simulink model "V2x_TC_CarBreakdownWarning_cs"  (Simulink 7.6)
settings: Solver=ode5  SolverMode=SingleTasking  StartTime=0.0  StopTime=18  FixedStep=1/100  RelTol=1e-3
PreLoadFcn:
  | check_NUTS_defined;
  | 
  | assignin('base',['model_closed_' bdroot],false);addpath('../includes_V2x');
InitFcn:
  | PreScanExperimentInitFcn(bdroot)
StopFcn:
  | PreScanExperimentStopFcn(bdroot)
undefined symbols (not defined in the file or in its folder): acceleration, actorID, actorType, DiscIntNeverNeededParam, GPS_alt, GPS_lat, GPS_long, intmax, lightBarInUse, messageID, Newton, publicActorType, Raphson, rotZ, sigbuilder_block, sireneInUse, trafficLightPriority, turnAdvice, velocity, x_ini_VRML, y_ini_VRML, yawRate, z_ini_VRML
libraries: simulink x61, PreScanSimulinkLibrary x19, PreScanUsefulBlocks x7, simulink_extras x1
(part 9 of 10)

== system V2x_TC_CarBreakdownWarning_cs/Audi_A8_1/Traffic Controller/Traffic signs and  traffic lights controller/Enabled Subsystem ==
  trafficSignType : Inport
  trafficLightsType : Inport  Port=2
  hostRotZ : Inport  Port=3
  hostVelocity : Inport  Port=4
  messageID : Inport  Port=5
  trafficLightPriority : Inport  Port=6
  rotZ : Inport  Port=7
  host GPS lat [deg] : Inport  Port=8
  host GPS long [deg] : Inport  Port=9
  host GPS alt [m] : Inport  Port=10
  GPS_lat : Inport  Port=11
  GPS_long : Inport  Port=12
  GPS_alt : Inport  Port=13
  Enable : EnablePort  StatesWhenEnabling=reset  PropagateVarSize=During execution
  GPS to XYZ difference (vectorized) : Subsystem
  Logical Operator : Logic  AllPortsSameDT=off  OutDataTypeStr=boolean
  Logical Operator1 : Logic  AllPortsSameDT=off  OutDataTypeStr=boolean
  Logical Operator2 : Logic  Inputs=4  AllPortsSameDT=off  OutDataTypeStr=boolean
  distance condition : Subsystem
  heading condition : Subsystem
  hostVelocity1 : InportShadow  Port=4
  major object selection lights : Subsystem
  major object selection signs : Subsystem
  orientation condition : Subsystem
  right road side condition : Subsystem
  signsWarning : Outport
  signsMessage : Outport  Port=2  InitialOutput=0
  lightsWarning : Outport  Port=3
  ligtsMessage : Outport  Port=4  InitialOutput=0
  ligtsPriority : Outport  Port=5  InitialOutput=0
  wires:
  GPS to XYZ difference (vectorized)/3(dY) -> right road side condition/3(dY), orientation condition/3(dY)
  right road side condition/1(orient_cond) -> Logical Operator2/4
  GPS to XYZ difference (vectorized)/1(dist_sq) -> distance condition/1(distance_squared)
  GPS to XYZ difference (vectorized)/2(dX) -> orientation condition/2(dX), right road side condition/2(dX)
  GPS to XYZ difference (vectorized)/4(dZ) -> orientation condition/4(dZ)
  GPS_alt/1 -> GPS to XYZ difference (vectorized)/6(alt)
  orientation condition/1(orient_cond) -> Logical Operator2/3
  GPS_long/1 -> GPS to XYZ difference (vectorized)/5(long)
  GPS_lat/1 -> GPS to XYZ difference (vectorized)/4(lat)
  host GPS alt [m]/1 -> GPS to XYZ difference (vectorized)/3(hostAlt)
  host GPS long [deg]/1 -> GPS to XYZ difference (vectorized)/2(hostLong)
  host GPS lat [deg]/1 -> GPS to XYZ difference (vectorized)/1(hostLat)
  hostVelocity1/1 -> major object selection signs/2(hostVelocity)
  major object selection lights/3(Priority) -> ligtsPriority/1
  major object selection lights/2(MessageID) -> ligtsMessage/1
  major object selection lights/1(Warning) -> lightsWarning/1
  trafficLightPriority/1 -> major object selection lights/3(traffic lights priorities)
  Logical Operator1/1 -> major object selection lights/1(conditions)
  major object selection signs/2(MessageID) -> signsMessage/1
  major object selection signs/1(Warning) -> signsWarning/1
  messageID/1 -> major object selection lights/2(messagesID), major object selection signs/3(messagesID)
  Logical Operator/1 -> major object selection signs/1(conditions)
  trafficLightsType/1 -> Logical Operator1/2
  trafficSignType/1 -> Logical Operator/2
  Logical Operator2/1 -> Logical Operator1/1, Logical Operator/1
  heading condition/1(head_cond) -> Logical Operator2/2
  distance condition/1(dist_cond) -> Logical Operator2/1
  hostRotZ/1 -> orientation condition/1(hostRotZ), right road side condition/1(hostRotZ), heading condition/1(hostRotZ)
  hostVelocity/1 -> distance condition/2(hostVelocity)
  rotZ/1 -> heading condition/2(rotZ)

== system V2x_TC_CarBreakdownWarning_cs/Audi_A8_1/Trajectories/Traj2State1/Traj2State2 ==
  traj : Inport
  MuxState : Subsystem
  Traj2MuxState_Ext : Subsystem
  state : Outport
  wires:
  Traj2MuxState_Ext/9(Y [rad]) -> MuxState/9(Y [rad])
  Traj2MuxState_Ext/8(P [rad]) -> MuxState/8(P [rad])
  Traj2MuxState_Ext/7(R [rad]) -> MuxState/7(R [rad])
  Traj2MuxState_Ext/6(dz [m/s]) -> MuxState/6(dz [m/s])
  Traj2MuxState_Ext/5(dy [m/s]) -> MuxState/5(dy [m/s])
  Traj2MuxState_Ext/4(dx [m/s]) -> MuxState/4(dx [m/s])
  Traj2MuxState_Ext/3(z [m]) -> MuxState/3(z [m])
  Traj2MuxState_Ext/2(y [m]) -> MuxState/2(y [m])
  Traj2MuxState_Ext/1(x [m]) -> MuxState/1(x [m])
  MuxState/1(state) -> state/1
  traj/1 -> Traj2MuxState_Ext/1(Traj)

== system V2x_TC_CarBreakdownWarning_cs/Audi_A8_1/Trajectories/Traj2State2/Traj2State2 ==
  traj : Inport
  MuxState : Subsystem
  Traj2MuxState_Ext : Subsystem
  state : Outport
  wires:
  Traj2MuxState_Ext/9(Y [rad]) -> MuxState/9(Y [rad])
  Traj2MuxState_Ext/8(P [rad]) -> MuxState/8(P [rad])
  Traj2MuxState_Ext/7(R [rad]) -> MuxState/7(R [rad])
  Traj2MuxState_Ext/6(dz [m/s]) -> MuxState/6(dz [m/s])
  Traj2MuxState_Ext/5(dy [m/s]) -> MuxState/5(dy [m/s])
  Traj2MuxState_Ext/4(dx [m/s]) -> MuxState/4(dx [m/s])
  Traj2MuxState_Ext/3(z [m]) -> MuxState/3(z [m])
  Traj2MuxState_Ext/2(y [m]) -> MuxState/2(y [m])
  Traj2MuxState_Ext/1(x [m]) -> MuxState/1(x [m])
  MuxState/1(state) -> state/1
  traj/1 -> Traj2MuxState_Ext/1(Traj)

== system V2x_TC_CarBreakdownWarning_cs/Audi_A8_1/vehicle CAM generator/CAM generation/maybe ==
  x [m] : Inport
  y [m] : Inport  Port=2
  z [m] : Inport  Port=3
  rotZ [deg] : Inport  Port=4
  velocity [m/s] : Inport  Port=5
  Action Port : ActionPort  PropagateVarSize=During execution  ActionType=else
  Add{,1..4} (5 alike) : Sum  Inputs=+-
  Add5 : Sum  Inputs=+++
  Compare To Constant : simulink/Logic and Bit Operations/Compare To Constant  SystemSampleTime=-1  relop=>  const=1  LogicOutDataTypeMode=uint8  ZeroCross=off
  Compare To Constant1 : simulink/Logic and Bit Operations/Compare To Constant  SystemSampleTime=-1  relop=>  const=4  LogicOutDataTypeMode=uint8  ZeroCross=off
  Compare To Constant2 : simulink/Logic and Bit Operations/Compare To Constant  SystemSampleTime=-1  relop=>  const=5^2  LogicOutDataTypeMode=uint8  ZeroCross=off
  Data Store Read : DataStoreRead  DataStoreName=CAM_velocity  SampleTime=0.01
  Data Store Read1 : DataStoreRead  DataStoreName=CAM_heading  SampleTime=0.01
  Data Store Read2 : DataStoreRead  DataStoreName=CAM_x  SampleTime=0.01
  Data Store Read3 : DataStoreRead  DataStoreName=CAM_y  SampleTime=0.01
  Data Store Read4 : DataStoreRead  DataStoreName=CAM_z  SampleTime=0.01
  If : If  IfExpression=u1
  If Action Subsystem : Subsystem  TreatAsAtomicUnit=on
  If Action Subsystem1 : Subsystem  TreatAsAtomicUnit=on
  Logical Operator : Logic  Operator=OR  Inputs=3  AllPortsSameDT=off  OutDataTypeStr=boolean
  Merge : Merge
  Product : Product  RndMeth=Zero
  Product1 : Product  RndMeth=Zero
  Product2 : Product  RndMeth=Zero
  rotZ [deg]1 : InportShadow  Port=4
  velocity [m/s]1 : InportShadow  Port=5
  x [m]1 : InportShadow  Port=1
  y [m]1 : InportShadow  Port=2
  z [m]1 : InportShadow  Port=3
  Out1 : Outport  OutputWhenDisabled=reset  InitialOutput=0
  wires:
  velocity [m/s]/1 -> Add/1
  Data Store Read/1 -> Add/2
  Add/1 -> Compare To Constant/1
  Add1/1 -> Compare To Constant1/1
  rotZ [deg]/1 -> Add1/1
  Data Store Read1/1 -> Add1/2
  x [m]/1 -> Add3/1
  Data Store Read2/1 -> Add3/2
  y [m]/1 -> Add2/1
  Data Store Read3/1 -> Add2/2
  z [m]/1 -> Add4/1
  Data Store Read4/1 -> Add4/2
  Add4/1 -> Product2/2, Product2/1
  Add2/1 -> Product1/2, Product1/1
  Add3/1 -> Product/2, Product/1
  Product/1 -> Add5/1
  Product1/1 -> Add5/2
  Product2/1 -> Add5/3
  Add5/1 -> Compare To Constant2/1
  Compare To Constant/1 -> Logical Operator/1
  Compare To Constant1/1 -> Logical Operator/2
  Compare To Constant2/1 -> Logical Operator/3
  Logical Operator/1 -> If/1
  If/1 -> If Action Subsystem/Action
  If/2 -> If Action Subsystem1/Action
  If Action Subsystem/1(Out1) -> Merge/1
  If Action Subsystem1/1(Out1) -> Merge/2
  Merge/1 -> Out1/1
  x [m]1/1 -> If Action Subsystem/1(x [m])
  y [m]1/1 -> If Action Subsystem/2(y [m])
  z [m]1/1 -> If Action Subsystem/3(z [m])
  rotZ [deg]1/1 -> If Action Subsystem/4(rotZ [deg])
  velocity [m/s]1/1 -> If Action Subsystem/5(velocity [m/s])

== system V2x_TC_CarBreakdownWarning_cs/Audi_A8_1/vehicle CAM generator/CAM generation/no ==
  Action Port : ActionPort  PropagateVarSize=During execution  ActionType=elseif
  Constant : Constant  Value=0
  Out1 : Outport  OutputWhenDisabled=reset  InitialOutput=0
  wires:
  Constant/1 -> Out1/1

== system V2x_TC_CarBreakdownWarning_cs/Audi_A8_1/vehicle CAM generator/CAM generation/yes ==
  x [m] : Inport
  y [m] : Inport  Port=2
  z [m] : Inport  Port=3
  rotZ [deg] : Inport  Port=4
  velocity [m/s] : Inport  Port=5
  Action Port : ActionPort  PropagateVarSize=During execution  ActionType=then
  Constant : Constant
  Data Store Write : DataStoreWrite  DataStoreName=CAM_velocity
  Data Store Write1 : DataStoreWrite  DataStoreName=CAM_heading
  Data Store Write2 : DataStoreWrite  DataStoreName=CAM_x
  Data Store Write3 : DataStoreWrite  DataStoreName=CAM_y
  Data Store Write4 : DataStoreWrite  DataStoreName=CAM_z
  Data Store Write5 : DataStoreWrite  DataStoreName=CAM_time
  Digital Clock1 : DigitalClock  SampleTime=0.01
  Out1 : Outport  OutputWhenDisabled=reset  InitialOutput=0
  wires:
  Constant/1 -> Out1/1
  velocity [m/s]/1 -> Data Store Write/1
  rotZ [deg]/1 -> Data Store Write1/1
  x [m]/1 -> Data Store Write2/1
  y [m]/1 -> Data Store Write3/1
  z [m]/1 -> Data Store Write4/1
  Digital Clock1/1 -> Data Store Write5/1

== system V2x_TC_CarBreakdownWarning_cs/Audi_A8_1/vehicle CAM generator/Subsystem/GPS Noise ==
  GPS_Noise_src : Inport
  Band-Limited White Noise1 : simulink/Sources/Band-Limited White Noise  SystemSampleTime=-1  Cov=1.7  Ts=0.01  seed=randi(intmax, 1)
  Constant : Constant  Value=1/(360*44)
  Product : Product  Inputs=3  RndMeth=Zero
  GPS_Noise : Outport
  wires:
  GPS_Noise_src/1 -> Product/1
  Band-Limited White Noise1/1 -> Product/2
  Constant/1 -> Product/3
  Product/1 -> GPS_Noise/1

== system V2x_TC_CarBreakdownWarning_cs/Audi_A8_1/vehicle CAM generator/Subsystem1/GPS Noise ==
  GPS_Noise_src : Inport
  Band-Limited White Noise1 : simulink/Sources/Band-Limited White Noise  SystemSampleTime=-1  Cov=1.7  Ts=0.01  seed=randi(intmax, 1)
  Constant : Constant  Value=1/(360*44)
  Product : Product  Inputs=3  RndMeth=Zero
  GPS_Noise : Outport
  wires:
  Product/1 -> GPS_Noise/1
  Constant/1 -> Product/3
  Band-Limited White Noise1/1 -> Product/2
  GPS_Noise_src/1 -> Product/1

== system V2x_TC_CarBreakdownWarning_cs/Audi_A8_1/vehicle CAM generator/Subsystem2/GPS Noise ==
  GPS_Noise_src : Inport
  Band-Limited White Noise1 : simulink/Sources/Band-Limited White Noise  SystemSampleTime=-1  Cov=1.7  Ts=0.01  seed=randi(intmax, 1)
  Constant : Constant  Value=1/(360*44)
  Product : Product  Inputs=3  RndMeth=Zero
  GPS_Noise : Outport
  wires:
  GPS_Noise_src/1 -> Product/1
  Band-Limited White Noise1/1 -> Product/2
  Constant/1 -> Product/3
  Product/1 -> GPS_Noise/1

== system V2x_TC_CarBreakdownWarning_cs/Audi_A8_1/vehicle CAM generator/Subsystem3/GPS Noise ==
  GPS_Noise_src : Inport
  Band-Limited White Noise1 : simulink/Sources/Band-Limited White Noise  SystemSampleTime=-1  Cov=1.7  Ts=0.01  seed=randi(intmax, 1)
  Constant : Constant  Value=1/(360*44)
  Product : Product  Inputs=3  RndMeth=Zero
  GPS_Noise : Outport
  wires:
  Product/1 -> GPS_Noise/1
  Constant/1 -> Product/3
  Band-Limited White Noise1/1 -> Product/2
  GPS_Noise_src/1 -> Product/1

== system V2x_TC_CarBreakdownWarning_cs/BMW_X5_1/SELF_Demux/compas converter/cart2compas ==
  Angle [deg] : Inport
  Constant : Constant  Value=90
  Constant1 : Constant  Value=360
  Gain : Gain  Gain=1/360
  Gain1 : Gain  Gain=360
  Gain2 : Gain  Gain=-1
  Rounding Function : Rounding
  Sum : Sum  Inputs=|-+
  Sum1 : Sum  Inputs=-+|
  Sum2 : Sum  Inputs=++|
  heading [deg] : Outport
  wires:
  Sum2/1 -> heading [deg]/1
  Constant1/1 -> Sum2/1
  Gain2/1 -> Sum2/2
  Constant/1 -> Sum1/1
  Sum1/1 -> Sum/2, Gain/1
  Sum/1 -> Gain2/1
  Angle [deg]/1 -> Sum1/2
  Gain1/1 -> Sum/1
  Rounding Function/1 -> Gain1/1
  Gain/1 -> Rounding Function/1

== system V2x_TC_CarBreakdownWarning_cs/BMW_X5_1/Trajectories/Traj2State1/Traj2State2 ==
  traj : Inport
  MuxState : Subsystem
  Traj2MuxState_Ext : Subsystem
  state : Outport
  wires:
  Traj2MuxState_Ext/9(Y [rad]) -> MuxState/9(Y [rad])
  Traj2MuxState_Ext/8(P [rad]) -> MuxState/8(P [rad])
  Traj2MuxState_Ext/7(R [rad]) -> MuxState/7(R [rad])
  Traj2MuxState_Ext/6(dz [m/s]) -> MuxState/6(dz [m/s])
  Traj2MuxState_Ext/5(dy [m/s]) -> MuxState/5(dy [m/s])
  Traj2MuxState_Ext/4(dx [m/s]) -> MuxState/4(dx [m/s])
  Traj2MuxState_Ext/3(z [m]) -> MuxState/3(z [m])
  Traj2MuxState_Ext/2(y [m]) -> MuxState/2(y [m])
  Traj2MuxState_Ext/1(x [m]) -> MuxState/1(x [m])
  MuxState/1(state) -> state/1
  traj/1 -> Traj2MuxState_Ext/1(Traj)

== system V2x_TC_CarBreakdownWarning_cs/BMW_X5_1/vehicle CAM generator/CAM generation/maybe ==
  x [m] : Inport
  y [m] : Inport  Port=2
  z [m] : Inport  Port=3
  rotZ [deg] : Inport  Port=4
  velocity [m/s] : Inport  Port=5
  Action Port : ActionPort  PropagateVarSize=During execution  ActionType=else
  Add{,1..4} (5 alike) : Sum  Inputs=+-
  Add5 : Sum  Inputs=+++
  Compare To Constant : simulink/Logic and Bit Operations/Compare To Constant  SystemSampleTime=-1  relop=>  const=1  LogicOutDataTypeMode=uint8  ZeroCross=off
  Compare To Constant1 : simulink/Logic and Bit Operations/Compare To Constant  SystemSampleTime=-1  relop=>  const=4  LogicOutDataTypeMode=uint8  ZeroCross=off
  Compare To Constant2 : simulink/Logic and Bit Operations/Compare To Constant  SystemSampleTime=-1  relop=>  const=5^2  LogicOutDataTypeMode=uint8  ZeroCross=off
  Data Store Read : DataStoreRead  DataStoreName=CAM_velocity  SampleTime=0.01
  Data Store Read1 : DataStoreRead  DataStoreName=CAM_heading  SampleTime=0.01
  Data Store Read2 : DataStoreRead  DataStoreName=CAM_x  SampleTime=0.01
  Data Store Read3 : DataStoreRead  DataStoreName=CAM_y  SampleTime=0.01
  Data Store Read4 : DataStoreRead  DataStoreName=CAM_z  SampleTime=0.01
  If : If  IfExpression=u1
  If Action Subsystem : Subsystem  TreatAsAtomicUnit=on
  If Action Subsystem1 : Subsystem  TreatAsAtomicUnit=on
  Logical Operator : Logic  Operator=OR  Inputs=3  AllPortsSameDT=off  OutDataTypeStr=boolean
  Merge : Merge
  Product : Product  RndMeth=Zero
  Product1 : Product  RndMeth=Zero
  Product2 : Product  RndMeth=Zero
  rotZ [deg]1 : InportShadow  Port=4
  velocity [m/s]1 : InportShadow  Port=5
  x [m]1 : InportShadow  Port=1
  y [m]1 : InportShadow  Port=2
  z [m]1 : InportShadow  Port=3
  Out1 : Outport  OutputWhenDisabled=reset  InitialOutput=0
  wires:
  velocity [m/s]/1 -> Add/1
  Data Store Read/1 -> Add/2
  Add/1 -> Compare To Constant/1
  Add1/1 -> Compare To Constant1/1
  rotZ [deg]/1 -> Add1/1
  Data Store Read1/1 -> Add1/2
  x [m]/1 -> Add3/1
  Data Store Read2/1 -> Add3/2
  y [m]/1 -> Add2/1
  Data Store Read3/1 -> Add2/2
  z [m]/1 -> Add4/1
  Data Store Read4/1 -> Add4/2
  Add4/1 -> Product2/2, Product2/1
  Add2/1 -> Product1/2, Product1/1
  Add3/1 -> Product/2, Product/1
  Product/1 -> Add5/1
  Product1/1 -> Add5/2
  Product2/1 -> Add5/3
  Add5/1 -> Compare To Constant2/1
  Compare To Constant/1 -> Logical Operator/1
  Compare To Constant1/1 -> Logical Operator/2
  Compare To Constant2/1 -> Logical Operator/3
  Logical Operator/1 -> If/1
  If/1 -> If Action Subsystem/Action
  If/2 -> If Action Subsystem1/Action
  If Action Subsystem/1(Out1) -> Merge/1
  If Action Subsystem1/1(Out1) -> Merge/2
  Merge/1 -> Out1/1
  x [m]1/1 -> If Action Subsystem/1(x [m])
  y [m]1/1 -> If Action Subsystem/2(y [m])
  z [m]1/1 -> If Action Subsystem/3(z [m])
  rotZ [deg]1/1 -> If Action Subsystem/4(rotZ [deg])
  velocity [m/s]1/1 -> If Action Subsystem/5(velocity [m/s])

== system V2x_TC_CarBreakdownWarning_cs/BMW_X5_1/vehicle CAM generator/CAM generation/no ==
  Action Port : ActionPort  PropagateVarSize=During execution  ActionType=elseif
  Constant : Constant  Value=0
  Out1 : Outport  OutputWhenDisabled=reset  InitialOutput=0
  wires:
  Constant/1 -> Out1/1

== system V2x_TC_CarBreakdownWarning_cs/BMW_X5_1/vehicle CAM generator/CAM generation/yes ==
  x [m] : Inport
  y [m] : Inport  Port=2
  z [m] : Inport  Port=3
  rotZ [deg] : Inport  Port=4
  velocity [m/s] : Inport  Port=5
  Action Port : ActionPort  PropagateVarSize=During execution  ActionType=then
  Constant : Constant
  Data Store Write : DataStoreWrite  DataStoreName=CAM_velocity
  Data Store Write1 : DataStoreWrite  DataStoreName=CAM_heading
  Data Store Write2 : DataStoreWrite  DataStoreName=CAM_x
  Data Store Write3 : DataStoreWrite  DataStoreName=CAM_y
  Data Store Write4 : DataStoreWrite  DataStoreName=CAM_z
  Data Store Write5 : DataStoreWrite  DataStoreName=CAM_time
  Digital Clock1 : DigitalClock  SampleTime=0.01
  Out1 : Outport  OutputWhenDisabled=reset  InitialOutput=0
  wires:
  Constant/1 -> Out1/1
  velocity [m/s]/1 -> Data Store Write/1
  rotZ [deg]/1 -> Data Store Write1/1
  x [m]/1 -> Data Store Write2/1
  y [m]/1 -> Data Store Write3/1
  z [m]/1 -> Data Store Write4/1
  Digital Clock1/1 -> Data Store Write5/1

== system V2x_TC_CarBreakdownWarning_cs/CameraTrolley/SELF_Demux/compas converter/cart2compas ==
  Angle [deg] : Inport
  Constant : Constant  Value=90
  Constant1 : Constant  Value=360
  Gain : Gain  Gain=1/360
  Gain1 : Gain  Gain=360
  Gain2 : Gain  Gain=-1
  Rounding Function : Rounding
  Sum : Sum  Inputs=|-+
  Sum1 : Sum  Inputs=-+|
  Sum2 : Sum  Inputs=++|
  heading [deg] : Outport
  wires:
  Sum2/1 -> heading [deg]/1
  Constant1/1 -> Sum2/1
  Gain2/1 -> Sum2/2
  Constant/1 -> Sum1/1
  Sum1/1 -> Sum/2, Gain/1
  Sum/1 -> Gain2/1
  Angle [deg]/1 -> Sum1/2
  Gain1/1 -> Sum/1
  Rounding Function/1 -> Gain1/1
  Gain/1 -> Rounding Function/1

== system V2x_TC_CarBreakdownWarning_cs/Fiat_Bravo_1/SELF_Demux/compas converter/cart2compas ==
  Angle [deg] : Inport
  Constant : Constant  Value=90
  Constant1 : Constant  Value=360
  Gain : Gain  Gain=1/360
  Gain1 : Gain  Gain=360
  Gain2 : Gain  Gain=-1
  Rounding Function : Rounding
  Sum : Sum  Inputs=|-+
  Sum1 : Sum  Inputs=-+|
  Sum2 : Sum  Inputs=++|
  heading [deg] : Outport
  wires:
  Sum2/1 -> heading [deg]/1
  Constant1/1 -> Sum2/1
  Gain2/1 -> Sum2/2
  Constant/1 -> Sum1/1
  Sum1/1 -> Sum/2, Gain/1
  Sum/1 -> Gain2/1
  Angle [deg]/1 -> Sum1/2
  Gain1/1 -> Sum/1
  Rounding Function/1 -> Gain1/1
  Gain/1 -> Rounding Function/1

== system V2x_TC_CarBreakdownWarning_cs/Fiat_Bravo_1/Trajectories/Traj2State1/Traj2State2 ==
  traj : Inport
  MuxState : Subsystem
  Traj2MuxState_Ext : Subsystem
  state : Outport
  wires:
  Traj2MuxState_Ext/9(Y [rad]) -> MuxState/9(Y [rad])
  Traj2MuxState_Ext/8(P [rad]) -> MuxState/8(P [rad])
  Traj2MuxState_Ext/7(R [rad]) -> MuxState/7(R [rad])
  Traj2MuxState_Ext/6(dz [m/s]) -> MuxState/6(dz [m/s])
  Traj2MuxState_Ext/5(dy [m/s]) -> MuxState/5(dy [m/s])
  Traj2MuxState_Ext/4(dx [m/s]) -> MuxState/4(dx [m/s])
  Traj2MuxState_Ext/3(z [m]) -> MuxState/3(z [m])
  Traj2MuxState_Ext/2(y [m]) -> MuxState/2(y [m])
  Traj2MuxState_Ext/1(x [m]) -> MuxState/1(x [m])
  MuxState/1(state) -> state/1
  traj/1 -> Traj2MuxState_Ext/1(Traj)

== system V2x_TC_CarBreakdownWarning_cs/Fiat_Bravo_1/vehicle CAM generator/CAM generation/maybe ==
  x [m] : Inport
  y [m] : Inport  Port=2
  z [m] : Inport  Port=3
  rotZ [deg] : Inport  Port=4
  velocity [m/s] : Inport  Port=5
  Action Port : ActionPort  PropagateVarSize=During execution  ActionType=else
  Add{,1..4} (5 alike) : Sum  Inputs=+-
  Add5 : Sum  Inputs=+++
  Compare To Constant : simulink/Logic and Bit Operations/Compare To Constant  SystemSampleTime=-1  relop=>  const=1  LogicOutDataTypeMode=uint8  ZeroCross=off
  Compare To Constant1 : simulink/Logic and Bit Operations/Compare To Constant  SystemSampleTime=-1  relop=>  const=4  LogicOutDataTypeMode=uint8  ZeroCross=off
  Compare To Constant2 : simulink/Logic and Bit Operations/Compare To Constant  SystemSampleTime=-1  relop=>  const=5^2  LogicOutDataTypeMode=uint8  ZeroCross=off
  Data Store Read : DataStoreRead  DataStoreName=CAM_velocity  SampleTime=0.01
  Data Store Read1 : DataStoreRead  DataStoreName=CAM_heading  SampleTime=0.01
  Data Store Read2 : DataStoreRead  DataStoreName=CAM_x  SampleTime=0.01
  Data Store Read3 : DataStoreRead  DataStoreName=CAM_y  SampleTime=0.01
  Data Store Read4 : DataStoreRead  DataStoreName=CAM_z  SampleTime=0.01
  If : If  IfExpression=u1
  If Action Subsystem : Subsystem  TreatAsAtomicUnit=on
  If Action Subsystem1 : Subsystem  TreatAsAtomicUnit=on
  Logical Operator : Logic  Operator=OR  Inputs=3  AllPortsSameDT=off  OutDataTypeStr=boolean
  Merge : Merge
  Product : Product  RndMeth=Zero
  Product1 : Product  RndMeth=Zero
  Product2 : Product  RndMeth=Zero
  rotZ [deg]1 : InportShadow  Port=4
  velocity [m/s]1 : InportShadow  Port=5
  x [m]1 : InportShadow  Port=1
  y [m]1 : InportShadow  Port=2
  z [m]1 : InportShadow  Port=3
  Out1 : Outport  OutputWhenDisabled=reset  InitialOutput=0
  wires:
  velocity [m/s]/1 -> Add/1
  Data Store Read/1 -> Add/2
  Add/1 -> Compare To Constant/1
  Add1/1 -> Compare To Constant1/1
  rotZ [deg]/1 -> Add1/1
  Data Store Read1/1 -> Add1/2
  x [m]/1 -> Add3/1
  Data Store Read2/1 -> Add3/2
  y [m]/1 -> Add2/1
  Data Store Read3/1 -> Add2/2
  z [m]/1 -> Add4/1
  Data Store Read4/1 -> Add4/2
  Add4/1 -> Product2/2, Product2/1
  Add2/1 -> Product1/2, Product1/1
  Add3/1 -> Product/2, Product/1
  Product/1 -> Add5/1
  Product1/1 -> Add5/2
  Product2/1 -> Add5/3
  Add5/1 -> Compare To Constant2/1
  Compare To Constant/1 -> Logical Operator/1
  Compare To Constant1/1 -> Logical Operator/2
  Compare To Constant2/1 -> Logical Operator/3
  Logical Operator/1 -> If/1
  If/1 -> If Action Subsystem/Action
  If/2 -> If Action Subsystem1/Action
  If Action Subsystem/1(Out1) -> Merge/1
  If Action Subsystem1/1(Out1) -> Merge/2
  Merge/1 -> Out1/1
  x [m]1/1 -> If Action Subsystem/1(x [m])
  y [m]1/1 -> If Action Subsystem/2(y [m])
  z [m]1/1 -> If Action Subsystem/3(z [m])
  rotZ [deg]1/1 -> If Action Subsystem/4(rotZ [deg])
  velocity [m/s]1/1 -> If Action Subsystem/5(velocity [m/s])

== system V2x_TC_CarBreakdownWarning_cs/Fiat_Bravo_1/vehicle CAM generator/CAM generation/no ==
  Action Port : ActionPort  PropagateVarSize=During execution  ActionType=elseif
  Constant : Constant  Value=0
  Out1 : Outport  OutputWhenDisabled=reset  InitialOutput=0
  wires:
  Constant/1 -> Out1/1

== system V2x_TC_CarBreakdownWarning_cs/Fiat_Bravo_1/vehicle CAM generator/CAM generation/yes ==
  x [m] : Inport
  y [m] : Inport  Port=2
  z [m] : Inport  Port=3
  rotZ [deg] : Inport  Port=4
  velocity [m/s] : Inport  Port=5
  Action Port : ActionPort  PropagateVarSize=During execution  ActionType=then
  Constant : Constant
  Data Store Write : DataStoreWrite  DataStoreName=CAM_velocity
  Data Store Write1 : DataStoreWrite  DataStoreName=CAM_heading
  Data Store Write2 : DataStoreWrite  DataStoreName=CAM_x
  Data Store Write3 : DataStoreWrite  DataStoreName=CAM_y
  Data Store Write4 : DataStoreWrite  DataStoreName=CAM_z
  Data Store Write5 : DataStoreWrite  DataStoreName=CAM_time
  Digital Clock1 : DigitalClock  SampleTime=0.01
  Out1 : Outport  OutputWhenDisabled=reset  InitialOutput=0
  wires:
  Constant/1 -> Out1/1
  velocity [m/s]/1 -> Data Store Write/1
  rotZ [deg]/1 -> Data Store Write1/1
  x [m]/1 -> Data Store Write2/1
  y [m]/1 -> Data Store Write3/1
  z [m]/1 -> Data Store Write4/1
  Digital Clock1/1 -> Data Store Write5/1

== system V2x_TC_CarBreakdownWarning_cs/Toyota_Previa_1/Antenna_Rx_1_Demux/compas converter/cart2compas ==
  Angle [deg] : Inport
  Constant : Constant  Value=90
  Constant1 : Constant  Value=360
  Gain : Gain  Gain=1/360
  Gain1 : Gain  Gain=360
  Gain2 : Gain  Gain=-1
  Rounding Function : Rounding
  Sum : Sum  Inputs=|-+
  Sum1 : Sum  Inputs=-+|
  Sum2 : Sum  Inputs=++|
  heading [deg] : Outport
  wires:
  Gain/1 -> Rounding Function/1
  Rounding Function/1 -> Gain1/1
  Gain1/1 -> Sum/1
  Angle [deg]/1 -> Sum1/2
  Sum/1 -> Gain2/1
  Sum1/1 -> Gain/1, Sum/2
  Constant/1 -> Sum1/1
  Gain2/1 -> Sum2/2
  Constant1/1 -> Sum2/1
  Sum2/1 -> heading [deg]/1

== system V2x_TC_CarBreakdownWarning_cs/Toyota_Previa_1/SELF_Demux/compas converter/cart2compas ==
  Angle [deg] : Inport
  Constant : Constant  Value=90
  Constant1 : Constant  Value=360
  Gain : Gain  Gain=1/360
  Gain1 : Gain  Gain=360
  Gain2 : Gain  Gain=-1
  Rounding Function : Rounding
  Sum : Sum  Inputs=|-+
  Sum1 : Sum  Inputs=-+|
  Sum2 : Sum  Inputs=++|
  heading [deg] : Outport
  wires:
  Sum2/1 -> heading [deg]/1
  Constant1/1 -> Sum2/1
  Gain2/1 -> Sum2/2
  Constant/1 -> Sum1/1
  Sum1/1 -> Sum/2, Gain/1
  Sum/1 -> Gain2/1
  Angle [deg]/1 -> Sum1/2
  Gain1/1 -> Sum/1
  Rounding Function/1 -> Gain1/1
  Gain/1 -> Rounding Function/1

== system V2x_TC_CarBreakdownWarning_cs/Toyota_Previa_1/vehicle CAM generator/CAM generation/maybe ==
  x [m] : Inport
  y [m] : Inport  Port=2
  z [m] : Inport  Port=3
  rotZ [deg] : Inport  Port=4
  velocity [m/s] : Inport  Port=5
  Action Port : ActionPort  PropagateVarSize=During execution  ActionType=else
  Add{,1..4} (5 alike) : Sum  Inputs=+-
  Add5 : Sum  Inputs=+++
  Compare To Constant : simulink/Logic and Bit Operations/Compare To Constant  SystemSampleTime=-1  relop=>  const=1  LogicOutDataTypeMode=uint8  ZeroCross=off
  Compare To Constant1 : simulink/Logic and Bit Operations/Compare To Constant  SystemSampleTime=-1  relop=>  const=4  LogicOutDataTypeMode=uint8  ZeroCross=off
  Compare To Constant2 : simulink/Logic and Bit Operations/Compare To Constant  SystemSampleTime=-1  relop=>  const=5^2  LogicOutDataTypeMode=uint8  ZeroCross=off
  Data Store Read : DataStoreRead  DataStoreName=CAM_velocity  SampleTime=0.01
  Data Store Read1 : DataStoreRead  DataStoreName=CAM_heading  SampleTime=0.01
  Data Store Read2 : DataStoreRead  DataStoreName=CAM_x  SampleTime=0.01
  Data Store Read3 : DataStoreRead  DataStoreName=CAM_y  SampleTime=0.01
  Data Store Read4 : DataStoreRead  DataStoreName=CAM_z  SampleTime=0.01
  If : If  IfExpression=u1
  If Action Subsystem : Subsystem  TreatAsAtomicUnit=on
  If Action Subsystem1 : Subsystem  TreatAsAtomicUnit=on
  Logical Operator : Logic  Operator=OR  Inputs=3  AllPortsSameDT=off  OutDataTypeStr=boolean
  Merge : Merge
  Product : Product  RndMeth=Zero
  Product1 : Product  RndMeth=Zero
  Product2 : Product  RndMeth=Zero
  rotZ [deg]1 : InportShadow  Port=4
  velocity [m/s]1 : InportShadow  Port=5
  x [m]1 : InportShadow  Port=1
  y [m]1 : InportShadow  Port=2
  z [m]1 : InportShadow  Port=3
  Out1 : Outport  OutputWhenDisabled=reset  InitialOutput=0
  wires:
  velocity [m/s]/1 -> Add/1
  Data Store Read/1 -> Add/2
  Add/1 -> Compare To Constant/1
  Add1/1 -> Compare To Constant1/1
  rotZ [deg]/1 -> Add1/1
  Data Store Read1/1 -> Add1/2
  x [m]/1 -> Add3/1
  Data Store Read2/1 -> Add3/2
  y [m]/1 -> Add2/1
  Data Store Read3/1 -> Add2/2
  z [m]/1 -> Add4/1
  Data Store Read4/1 -> Add4/2
  Add4/1 -> Product2/2, Product2/1
  Add2/1 -> Product1/2, Product1/1
  Add3/1 -> Product/2, Product/1
  Product/1 -> Add5/1
  Product1/1 -> Add5/2
  Product2/1 -> Add5/3
  Add5/1 -> Compare To Constant2/1
  Compare To Constant/1 -> Logical Operator/1
  Compare To Constant1/1 -> Logical Operator/2
  Compare To Constant2/1 -> Logical Operator/3
  Logical Operator/1 -> If/1
  If/1 -> If Action Subsystem/Action
  If/2 -> If Action Subsystem1/Action
  If Action Subsystem/1(Out1) -> Merge/1
  If Action Subsystem1/1(Out1) -> Merge/2
  Merge/1 -> Out1/1
  x [m]1/1 -> If Action Subsystem/1(x [m])
  y [m]1/1 -> If Action Subsystem/2(y [m])
  z [m]1/1 -> If Action Subsystem/3(z [m])
  rotZ [deg]1/1 -> If Action Subsystem/4(rotZ [deg])
  velocity [m/s]1/1 -> If Action Subsystem/5(velocity [m/s])

== system V2x_TC_CarBreakdownWarning_cs/Toyota_Previa_1/vehicle CAM generator/CAM generation/no ==
  Action Port : ActionPort  PropagateVarSize=During execution  ActionType=elseif
  Constant : Constant  Value=0
  Out1 : Outport  OutputWhenDisabled=reset  InitialOutput=0
  wires:
  Constant/1 -> Out1/1

== system V2x_TC_CarBreakdownWarning_cs/Toyota_Previa_1/vehicle CAM generator/CAM generation/yes ==
  x [m] : Inport
  y [m] : Inport  Port=2
  z [m] : Inport  Port=3
  rotZ [deg] : Inport  Port=4
  velocity [m/s] : Inport  Port=5
  Action Port : ActionPort  PropagateVarSize=During execution  ActionType=then
  Constant : Constant
  Data Store Write : DataStoreWrite  DataStoreName=CAM_velocity
  Data Store Write1 : DataStoreWrite  DataStoreName=CAM_heading
  Data Store Write2 : DataStoreWrite  DataStoreName=CAM_x
  Data Store Write3 : DataStoreWrite  DataStoreName=CAM_y
  Data Store Write4 : DataStoreWrite  DataStoreName=CAM_z
  Data Store Write5 : DataStoreWrite  DataStoreName=CAM_time
  Digital Clock1 : DigitalClock  SampleTime=0.01
  Out1 : Outport  OutputWhenDisabled=reset  InitialOutput=0
  wires:
  Constant/1 -> Out1/1
  velocity [m/s]/1 -> Data Store Write/1
  rotZ [deg]/1 -> Data Store Write1/1
  x [m]/1 -> Data Store Write2/1
  y [m]/1 -> Data Store Write3/1
  z [m]/1 -> Data Store Write4/1
  Digital Clock1/1 -> Data Store Write5/1

== system V2x_TC_CarBreakdownWarning_cs/Toyota_Previa_1/vehicle CAM generator/Subsystem/GPS Noise ==
  GPS_Noise_src : Inport
  Band-Limited White Noise1 : simulink/Sources/Band-Limited White Noise  SystemSampleTime=-1  Cov=1.7  Ts=0.01  seed=randi(intmax, 1)
  Constant : Constant  Value=1/(360*44)
  Product : Product  Inputs=3  RndMeth=Zero
  GPS_Noise : Outport
  wires:
  GPS_Noise_src/1 -> Product/1
  Band-Limited White Noise1/1 -> Product/2
  Constant/1 -> Product/3
  Product/1 -> GPS_Noise/1

== system V2x_TC_CarBreakdownWarning_cs/Toyota_Previa_1/vehicle CAM generator/Subsystem1/GPS Noise ==
  GPS_Noise_src : Inport
  Band-Limited White Noise1 : simulink/Sources/Band-Limited White Noise  SystemSampleTime=-1  Cov=1.7  Ts=0.01  seed=randi(intmax, 1)
  Constant : Constant  Value=1/(360*44)
  Product : Product  Inputs=3  RndMeth=Zero
  GPS_Noise : Outport
  wires:
  Product/1 -> GPS_Noise/1
  Constant/1 -> Product/3
  Band-Limited White Noise1/1 -> Product/2
  GPS_Noise_src/1 -> Product/1

== system V2x_TC_CarBreakdownWarning_cs/Toyota_Previa_1/vehicle CAM generator/Subsystem2/GPS Noise ==
  GPS_Noise_src : Inport
  Band-Limited White Noise1 : simulink/Sources/Band-Limited White Noise  SystemSampleTime=-1  Cov=1.7  Ts=0.01  seed=randi(intmax, 1)
  Constant : Constant  Value=1/(360*44)
  Product : Product  Inputs=3  RndMeth=Zero
  GPS_Noise : Outport
  wires:
  GPS_Noise_src/1 -> Product/1
  Band-Limited White Noise1/1 -> Product/2
  Constant/1 -> Product/3
  Product/1 -> GPS_Noise/1

== system V2x_TC_CarBreakdownWarning_cs/Toyota_Previa_1/vehicle CAM generator/Subsystem3/GPS Noise ==
  GPS_Noise_src : Inport
  Band-Limited White Noise1 : simulink/Sources/Band-Limited White Noise  SystemSampleTime=-1  Cov=1.7  Ts=0.01  seed=randi(intmax, 1)
  Constant : Constant  Value=1/(360*44)
  Product : Product  Inputs=3  RndMeth=Zero
  GPS_Noise : Outport
  wires:
  Product/1 -> GPS_Noise/1
  Constant/1 -> Product/3
  Band-Limited White Noise1/1 -> Product/2
  GPS_Noise_src/1 -> Product/1

== system V2x_TC_CarBreakdownWarning_cs/Audi_A8_1/Traffic Controller/Intersection warning controller/Enabled Subsystem/Intersection ==
  hostRotZ : Inport
  hostTurnAdvice : Inport  Port=2
  host GPS lat [deg] : Inport  Port=3
  host GPS long [deg] : Inport  Port=4
  host GPS alt [m] : Inport  Port=5
  GPS_lat : Inport  Port=6
  GPS_long : Inport  Port=7
  GPS_alt : Inport  Port=8
  targetVelocity : Inport  Port=9
  turnAdvice : Inport  Port=10
  rotZ : Inport  Port=11
  actorType : Inport  Port=12
  crossingType : Inport  Port=13
  crossing detection range : Inport  Port=14
  Closest crossing selection : Subsystem
  GPS to XYZ difference (vectorized) : Subsystem
  GPS_alt_1 : InportShadow  Port=8
  GPS_lat_1 : InportShadow  Port=6
  GPS_long_1 : InportShadow  Port=7
  Intersection collision warning controller : Subsystem
  Terminator_2 : Terminator
  cartesian 2 cylindrical : Subsystem
  crossing detection range_1 : InportShadow  Port=14
  hostRotZ_1 : InportShadow  Port=1
  relative heading : Subsystem
  warning left lane : Outport
  warning straight lane : Outport  Port=2
  warning right lane : Outport  Port=3
  wires:
  host GPS lat [deg]/1 -> Closest crossing selection/2(host GPS lat)
  host GPS long [deg]/1 -> Closest crossing selection/3(host GPS long)
  host GPS alt [m]/1 -> Closest crossing selection/4(host GPS alt)
  Closest crossing selection/1(crossing GPS lat) -> GPS to XYZ difference (vectorized)/1(hostLat)
  Closest crossing selection/2(crossing GPS long) -> GPS to XYZ difference (vectorized)/2(hostLong)
  Closest crossing selection/3(crossing GPS alt) -> GPS to XYZ difference (vectorized)/3(hostAlt)
  crossing detection range/1 -> Closest crossing selection/8(crossing detection range)
  crossing detection range_1/1 -> Intersection collision warning controller/3(crossing detection range)
  hostRotZ/1 -> relative heading/2(hostRotZ)
  hostTurnAdvice/1 -> Intersection collision warning controller/2(hostTurnAdvice)
  cartesian 2 cylindrical/1(range) -> Intersection collision warning controller/6(target range)
  relative heading/1(dRotZ) -> Intersection collision warning controller/8(target heading)
  Intersection collision warning controller/1(warning left lane) -> warning left lane/1
  Intersection collision warning controller/2(warning straight lane) -> warning straight lane/1
  Intersection collision warning controller/3(warning right lane) -> warning right lane/1
  GPS to XYZ difference (vectorized)/1(dX) -> cartesian 2 cylindrical/1(dX)
  GPS to XYZ difference (vectorized)/2(dY) -> cartesian 2 cylindrical/2(dY)
  GPS_lat/1 -> Closest crossing selection/5(GPS lat)
  GPS_long/1 -> Closest crossing selection/6(GPS long)
  GPS_alt/1 -> Closest crossing selection/7(GPS alt)
  crossingType/1 -> Closest crossing selection/1(crossingType)
  rotZ/1 -> relative heading/1(rotZ)
  GPS_lat_1/1 -> GPS to XYZ difference (vectorized)/4(lat)
  GPS_long_1/1 -> GPS to XYZ difference (vectorized)/5(long)
  GPS_alt_1/1 -> GPS to XYZ difference (vectorized)/6(alt)
  turnAdvice/1 -> Intersection collision warning controller/4(target intention)
  targetVelocity/1 -> Intersection collision warning controller/5(target velocity)
  actorType/1 -> Intersection collision warning controller/1(actorType)
  GPS to XYZ difference (vectorized)/3(dZ) -> Terminator_2/1
  hostRotZ_1/1 -> cartesian 2 cylindrical/3(hostRotZ)
  cartesian 2 cylindrical/2(angle) -> Intersection collision warning controller/7(target angle)

== system V2x_TC_CarBreakdownWarning_cs/Audi_A8_1/Traffic Controller/Intersection warning controller/Enabled Subsystem/sort using ID ==
  IDs : Inport
  in1 : Inport  Port=2
  in2 : Inport  Port=3
  in3 : Inport  Port=4
  in4 : Inport  Port=5
  in5 : Inport  Port=6
  in6 : Inport  Port=7
  in7 : Inport  Port=8
  in8 : Inport  Port=9
  Embedded MATLAB Function : Stateflow chart  TreatAsAtomicUnit=on
  Selector{1..8} (8 alike) : Selector  IndexOptions=Index vector (port)  Indices=[1 3]  OutputSizes=1
  Out1 : Outport
  Out2 : Outport  Port=2
  Out3 : Outport  Port=3
  Out4 : Outport  Port=4
  Out5 : Outport  Port=5
  Out6 : Outport  Port=6
  Out7 : Outport  Port=7
  Out8 : Outport  Port=8
  wires:
  Embedded MATLAB Function/1(y) -> Selector7/2, Selector8/2, Selector6/2, Selector5/2, Selector4/2, Selector3/2, Selector2/2, Selector1/2
  IDs/1 -> Embedded MATLAB Function/1(ids)
  in7/1 -> Selector7/1
  in6/1 -> Selector6/1
  Selector7/1 -> Out7/1
  Selector6/1 -> Out6/1
  in5/1 -> Selector5/1
  in4/1 -> Selector4/1
  in3/1 -> Selector3/1
  in2/1 -> Selector2/1
  Selector5/1 -> Out5/1
  Selector4/1 -> Out4/1
  Selector3/1 -> Out3/1
  Selector2/1 -> Out2/1
  Selector1/1 -> Out1/1
  in1/1 -> Selector1/1
  in8/1 -> Selector8/1
  Selector8/1 -> Out8/1

== system V2x_TC_CarBreakdownWarning_cs/Audi_A8_1/Traffic Controller/Road accident detection controller/Compute distance to road accident/If Action Subsystem ==
  conditions : Inport
  GPS lat1 : Inport  Port=2
  GPS long1 : Inport  Port=3
  GPS alt1 : Inport  Port=4
  host_GPS_lat : Inport  Port=5
  host_GPS_long : Inport  Port=6
  host_GPS_alt : Inport  Port=7
  Action Port : ActionPort  PropagateVarSize=During execution  ActionType=then
  GPS to distance : Subsystem
  Product7 : Product  RndMeth=Zero
  Product8 : Product  RndMeth=Zero
  Product9 : Product  RndMeth=Zero
  Sum6 : Sum  Inputs=+
  Sum7 : Sum  Inputs=+
  Sum8 : Sum  Inputs=+
  distance : Outport  InitialOutput=0
  wires:
  conditions/1 -> Product7/1, Product9/1, Product8/1
  GPS lat1/1 -> Product7/2
  GPS long1/1 -> Product8/2
  GPS alt1/1 -> Product9/2
  Product7/1 -> Sum6/1
  Product8/1 -> Sum7/1
  Product9/1 -> Sum8/1
  Sum6/1 -> GPS to distance/4(lat)
  Sum7/1 -> GPS to distance/5(long)
  Sum8/1 -> GPS to distance/6(alt)
  host_GPS_lat/1 -> GPS to distance/1(hostLat)
  host_GPS_long/1 -> GPS to distance/2(hostLong)
  host_GPS_alt/1 -> GPS to distance/3(hostAlt)
  GPS to distance/1(dist) -> distance/1

== system V2x_TC_CarBreakdownWarning_cs/Audi_A8_1/Traffic Controller/Road accident detection controller/Compute distance to road accident/If Action Subsystem1 ==
  Action Port : ActionPort  PropagateVarSize=During execution  ActionType=else
  Constant : Constant  Value=0
  distance : Outport  InitialOutput=0
  wires:
  Constant/1 -> distance/1

== system V2x_TC_CarBreakdownWarning_cs/Audi_A8_1/Traffic Controller/Traffic signs and  traffic lights controller/Enabled Subsystem/GPS to XYZ difference (vectorized) ==
  hostLat : Inport
  hostLong : Inport  Port=2
  hostAlt : Inport  Port=3
  lat : Inport  Port=4
  long : Inport  Port=5
  alt : Inport  Port=6
  Add : Sum  Inputs=+-
  Add1 : Sum  Inputs=+-
  Add2 : Sum  Inputs=+-
  Add3 : Sum  Inputs=+++
  Product{,1..4} (5 alike) : Product  RndMeth=Zero
  d2r : Gain  Gain=pi/180
  d2r1 : Gain  Gain=pi/180
  mean Earth radius (latitudal) : Constant  Value=6335439.8775
  mean Earth radius (longitudal) : Constant  Value=6378137.55
  dist_sq : Outport
  dX : Outport  Port=2
  dY : Outport  Port=3
  dZ : Outport  Port=4
  wires:
  Add3/1 -> dist_sq/1
  Product4/1 -> Add3/3
  Product3/1 -> Add3/2
  Product/1 -> Add3/1
  Add2/1 -> Product4/1, Product4/2, dZ/1
  Product1/1 -> Product3/2, Product3/1, dX/1
  Product2/1 -> Product/2, Product/1, dY/1
  mean Earth radius (latitudal)/1 -> Product2/2
  mean Earth radius (longitudal)/1 -> Product1/2
  d2r1/1 -> Product1/1
  d2r/1 -> Product2/1
  Add1/1 -> d2r1/1
  Add/1 -> d2r/1
  hostAlt/1 -> Add2/2
  alt/1 -> Add2/1
  hostLong/1 -> Add1/2
  long/1 -> Add1/1
  hostLat/1 -> Add/2
  lat/1 -> Add/1

== system V2x_TC_CarBreakdownWarning_cs/Audi_A8_1/Traffic Controller/Traffic signs and  traffic lights controller/Enabled Subsystem/distance condition ==
  distance_squared : Inport
  hostVelocity : Inport  Port=2
  If : If  IfExpression=u1 ~= 0
  If Action Subsystem : Subsystem  TreatAsAtomicUnit=on
  If Action Subsystem1 : Subsystem  TreatAsAtomicUnit=on
  Merge : Merge
  Product3 : Product  RndMeth=Zero
  Product4 : Product  RndMeth=Zero
  Relational Operator1 : RelationalOperator  Operator=<  OutDataTypeStr=boolean
  headway time : Constant  Value=3
  dist_cond : Outport
  wires:
  Product3/1 -> If Action Subsystem1/1(headway time), Relational Operator1/2
  distance_squared/1 -> If Action Subsystem1/2(d2), If Action Subsystem/1(d2)
  Relational Operator1/1 -> dist_cond/1
  Merge/1 -> Relational Operator1/1
  If Action Subsystem1/1(t2) -> Merge/2
  If Action Subsystem/1(t2) -> Merge/1
  Product4/1 -> If Action Subsystem/2(v2)
  If/2 -> If Action Subsystem1/Action
  If/1 -> If Action Subsystem/Action
  hostVelocity/1 -> Product4/2, Product4/1, If/1
  headway time/1 -> Product3/1, Product3/2

== system V2x_TC_CarBreakdownWarning_cs/Audi_A8_1/Traffic Controller/Traffic signs and  traffic lights controller/Enabled Subsystem/heading condition ==
  hostRotZ : Inport
  rotZ : Inport  Port=2
  Abs : Abs
  Add : Sum  Inputs=+-
  Add1 : Sum  Inputs=-+
  Bias : Bias  Bias=180
  Constant : Constant  Value=360
  Constant1 : Constant  Value=360
  Logical Operator : Logic  Operator=OR  AllPortsSameDT=off  OutDataTypeStr=boolean
  Math Function : Math  Operator=mod  SaturateOnIntegerOverflow=on
  Relational Operator : RelationalOperator  Operator=<  OutDataTypeStr=boolean
  Relational Operator1 : RelationalOperator  Operator=>  OutDataTypeStr=boolean
  heading difference : Constant  Value=45
  head_cond : Outport
  wires:
  Logical Operator/1 -> head_cond/1
  Relational Operator1/1 -> Logical Operator/2
  Relational Operator/1 -> Logical Operator/1
  Constant1/1 -> Add1/2
  Add1/1 -> Relational Operator1/2
  heading difference/1 -> Add1/1, Relational Operator/2
  Abs/1 -> Relational Operator1/1, Relational Operator/1
  Math Function/1 -> Abs/1
  hostRotZ/1 -> Add/2
  rotZ/1 -> Add/1
  Bias/1 -> Math Function/1
  Constant/1 -> Math Function/2
  Add/1 -> Bias/1

== system V2x_TC_CarBreakdownWarning_cs/Audi_A8_1/Traffic Controller/Traffic signs and  traffic lights controller/Enabled Subsystem/major object selection lights ==
  conditions : Inport
  messagesID : Inport  Port=2
  traffic lights priorities : Inport  Port=3
  If : If  IfExpression=u1
  If Action Subsystem : Subsystem  TreatAsAtomicUnit=on
  If Action Subsystem1 : Subsystem  TreatAsAtomicUnit=on
  Logical Operator1 : Logic  Operator=OR  Inputs=1  AllPortsSameDT=off  OutDataTypeStr=boolean
  Merge : Merge
  Merge2 : Merge
  Traffic Lights Warning : Subsystem
  Warning : Outport
  MessageID : Outport  Port=2
  Priority : Outport  Port=3
  wires:
  Traffic Lights Warning/1(Warning) -> Warning/1
  Merge/1 -> Traffic Lights Warning/1(trafficLightPriority), Priority/1
  Merge2/1 -> MessageID/1
  If Action Subsystem/2(Priority) -> Merge/1
  If Action Subsystem/1(Message) -> Merge2/1
  If Action Subsystem1/1(Message) -> Merge2/2
  If Action Subsystem1/2(Priority) -> Merge/2
  traffic lights priorities/1 -> If Action Subsystem/3(traffic lights priorities)
  messagesID/1 -> If Action Subsystem/2(messagesID)
  conditions/1 -> If Action Subsystem/1(cond), Logical Operator1/1
  If/2 -> If Action Subsystem1/Action
  If/1 -> If Action Subsystem/Action
  Logical Operator1/1 -> If/1

== system V2x_TC_CarBreakdownWarning_cs/Audi_A8_1/Traffic Controller/Traffic signs and  traffic lights controller/Enabled Subsystem/major object selection signs ==
  conditions : Inport
  hostVelocity : Inport  Port=2
  messagesID : Inport  Port=3
  If : If  IfExpression=u1
  If Action Subsystem : Subsystem  TreatAsAtomicUnit=on
  If Action Subsystem1 : Subsystem  TreatAsAtomicUnit=on
  Logical Operator1 : Logic  Operator=OR  Inputs=1  AllPortsSameDT=off  OutDataTypeStr=boolean
  Merge : Merge
  Merge1 : Merge
  Warning : Outport
  MessageID : Outport  Port=2
  wires:
  hostVelocity/1 -> If Action Subsystem/3(hostVelocity)
  Merge/1 -> MessageID/1
  Merge1/1 -> Warning/1
  If Action Subsystem1/1(Warning) -> Merge1/2
  If Action Subsystem/1(Warning) -> Merge1/1
  If Action Subsystem/2(Message) -> Merge/1
  If Action Subsystem1/2(Message) -> Merge/2
  messagesID/1 -> If Action Subsystem/2(messagesID)
  conditions/1 -> If Action Subsystem/1(cond), Logical Operator1/1
  If/2 -> If Action Subsystem1/Action
  If/1 -> If Action Subsystem/Action
  Logical Operator1/1 -> If/1

== system V2x_TC_CarBreakdownWarning_cs/Audi_A8_1/Traffic Controller/Traffic signs and  traffic lights controller/Enabled Subsystem/orientation condition ==
  hostRotZ : Inport
  dX : Inport  Port=2
  dY : Inport  Port=3
  dZ : Inport  Port=4
  Abs : Abs
  Gain : Gain  Gain=pi/180
  Relational Operator : RelationalOperator  Operator=<  OutDataTypeStr=boolean
  Terminator : Terminator
  Trigonometric Function : Trigonometry  Operator=atan2
  d2r : Gain  Gain=pi/180
  orientation limit : Constant  Value=45
  to local reference system : Subsystem
  orient_cond : Outport
  wires:
  to local reference system/2(dx) -> Trigonometric Function/2
  to local reference system/1(dy) -> Trigonometric Function/1
  dY/1 -> to local reference system/3(dY)
  dX/1 -> to local reference system/2(dX)
  Gain/1 -> to local reference system/1(rotZ)
  hostRotZ/1 -> Gain/1
  Trigonometric Function/1 -> Abs/1
  Relational Operator/1 -> orient_cond/1
  d2r/1 -> Relational Operator/2
  Abs/1 -> Relational Operator/1
  orientation limit/1 -> d2r/1
  dZ/1 -> Terminator/1

== system V2x_TC_CarBreakdownWarning_cs/Audi_A8_1/Traffic Controller/Traffic signs and  traffic lights controller/Enabled Subsystem/right road side condition ==
  hostRotZ : Inport
  dX : Inport  Port=2
  dY : Inport  Port=3
  Compare To Zero : simulink/Logic and Bit Operations/Compare To Zero  SystemSampleTime=-1  relop=<  LogicOutDataTypeMode=boolean
  Gain : Gain  Gain=pi/180
  to local reference system : Subsystem
  orient_cond : Outport
  wires:
  Compare To Zero/1 -> orient_cond/1
  hostRotZ/1 -> Gain/1
  Gain/1 -> to local reference system/1(rotZ)
  dX/1 -> to local reference system/2(dX)
  dY/1 -> to local reference system/3(dY)
  to local reference system/1(dy) -> Compare To Zero/1

== system V2x_TC_CarBreakdownWarning_cs/Audi_A8_1/Trajectories/Traj2State1/Traj2State2/MuxState ==
  x [m] : Inport
  y [m] : Inport  Port=2
  z [m] : Inport  Port=3
  dx [m/s] : Inport  Port=4
  dy [m/s] : Inport  Port=5
  dz [m/s] : Inport  Port=6
  R [rad] : Inport  Port=7
  P [rad] : Inport  Port=8
  Y [rad] : Inport  Port=9
  Mux : Mux  Inputs=9
  state : Outport
  wires:
  z [m]/1 -> Mux/3
  y [m]/1 -> Mux/2
  x [m]/1 -> Mux/1
  Y [rad]/1 -> Mux/9
  P [rad]/1 -> Mux/8
  R [rad]/1 -> Mux/7
  dz [m/s]/1 -> Mux/6
  dy [m/s]/1 -> Mux/5
  dx [m/s]/1 -> Mux/4
  Mux/1 -> state/1

== system V2x_TC_CarBreakdownWarning_cs/Audi_A8_1/Trajectories/Traj2State1/Traj2State2/Traj2MuxState_Ext ==
  Traj : Inport
  Terminator{1..9} (9 alike) : Terminator
  demux : Subsystem
  x [m] : Outport
  y [m] : Outport  Port=2
  z [m] : Outport  Port=3
  dx [m/s] : Outport  Port=4
  dy [m/s] : Outport  Port=5
  dz [m/s] : Outport  Port=6
  R [rad] : Outport  Port=7
  P [rad] : Outport  Port=8
  Y [rad] : Outport  Port=9
  wires:
  demux/9(Y) -> Y [rad]/1
  demux/7(R) -> R [rad]/1
  demux/5(vely) -> dy [m/s]/1
  demux/4(velx) -> dx [m/s]/1
  demux/10(velR) -> Terminator4/1
  demux/11(velP) -> Terminator5/1
  demux/12(velY) -> Terminator1/1
  demux/13(accx) -> Terminator8/1
  demux/14(accy) -> Terminator9/1
  demux/15(accz) -> Terminator7/1
  demux/18(accY) -> Terminator2/1
  demux/16(accR) -> Terminator3/1
  demux/17(accP) -> Terminator6/1
  demux/3(z) -> z [m]/1
  Traj/1 -> demux/1(traj)
  demux/6(velz) -> dz [m/s]/1
  demux/1(x) -> x [m]/1
  demux/2(y) -> y [m]/1
  demux/8(P) -> P [rad]/1

== system V2x_TC_CarBreakdownWarning_cs/Audi_A8_1/Trajectories/Traj2State2/Traj2State2/MuxState ==
  x [m] : Inport
  y [m] : Inport  Port=2
  z [m] : Inport  Port=3
  dx [m/s] : Inport  Port=4
  dy [m/s] : Inport  Port=5
  dz [m/s] : Inport  Port=6
  R [rad] : Inport  Port=7
  P [rad] : Inport  Port=8
  Y [rad] : Inport  Port=9
  Mux : Mux  Inputs=9
  state : Outport
  wires:
  z [m]/1 -> Mux/3
  y [m]/1 -> Mux/2
  x [m]/1 -> Mux/1
  Y [rad]/1 -> Mux/9
  P [rad]/1 -> Mux/8
  R [rad]/1 -> Mux/7
  dz [m/s]/1 -> Mux/6
  dy [m/s]/1 -> Mux/5
  dx [m/s]/1 -> Mux/4
  Mux/1 -> state/1

== system V2x_TC_CarBreakdownWarning_cs/Audi_A8_1/Trajectories/Traj2State2/Traj2State2/Traj2MuxState_Ext ==
  Traj : Inport
  Terminator{1..9} (9 alike) : Terminator
  demux : Subsystem
  x [m] : Outport
  y [m] : Outport  Port=2
  z [m] : Outport  Port=3
  dx [m/s] : Outport  Port=4
  dy [m/s] : Outport  Port=5
  dz [m/s] : Outport  Port=6
  R [rad] : Outport  Port=7
  P [rad] : Outport  Port=8
  Y [rad] : Outport  Port=9
  wires:
  demux/9(Y) -> Y [rad]/1
  demux/7(R) -> R [rad]/1
  demux/5(vely) -> dy [m/s]/1
  demux/4(velx) -> dx [m/s]/1
  demux/10(velR) -> Terminator4/1
  demux/11(velP) -> Terminator5/1
  demux/12(velY) -> Terminator1/1
  demux/13(accx) -> Terminator8/1
  demux/14(accy) -> Terminator9/1
  demux/15(accz) -> Terminator7/1
  demux/18(accY) -> Terminator2/1
  demux/16(accR) -> Terminator3/1
  demux/17(accP) -> Terminator6/1
  demux/3(z) -> z [m]/1
  Traj/1 -> demux/1(traj)
  demux/6(velz) -> dz [m/s]/1
  demux/1(x) -> x [m]/1
  demux/2(y) -> y [m]/1
  demux/8(P) -> P [rad]/1
